simulink model "nlin_1DOF"  (R2025a)
settings: Solver=VariableStepAuto  StartTime=0.0  StopTime=50  RelTol=1e-3
settings Model: Creator=jidki  LastModifiedBy=jidki

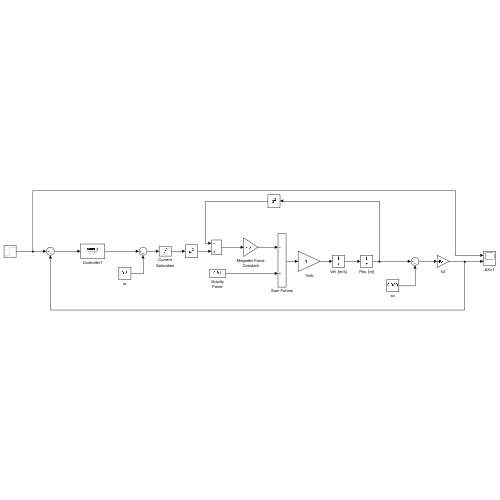
[thumbnail: Simulink's stored preview of the top-level diagram]
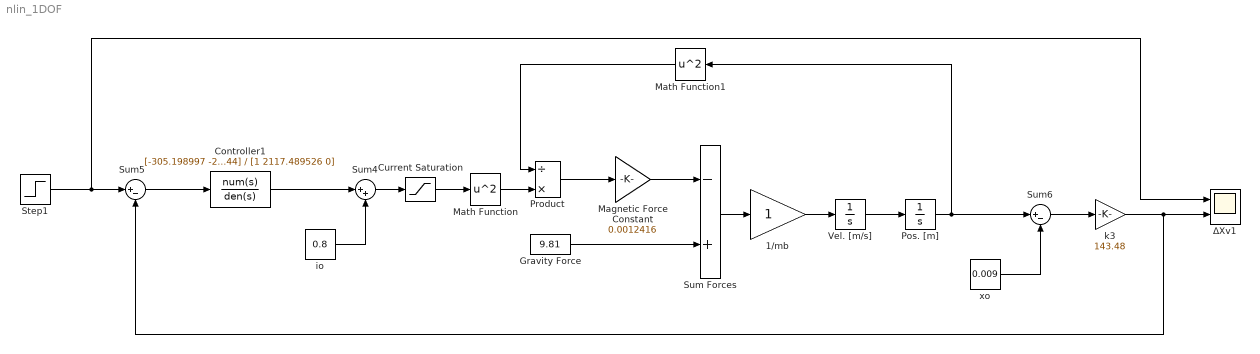
== system nlin_1DOF ==
  1/mb : Gain  SaturateOnIntegerOverflow=on  OutDataTypeStr=Inherit: Same as input  ParamDataTypeStr=Inherit: Same as input
  Controller1 : TransferFcn  Numerator=[-305.198997 -2531.996576 -2834.571544]  Denominator=[1 2117.489526 0]
  Current Saturation : Saturate  UpperLimit=1000  LowerLimit=-1000  ZeroCross=off
  Gravity Force : Constant  Value=9.81
  Magnetic Force Constant : Gain  Gain=0.0012416  SaturateOnIntegerOverflow=on  OutDataTypeStr=Inherit: Same as input  ParamDataTypeStr=Inherit: Same as input
  Math Function : Math  Operator=square  SignedPower=on
  Math Function1 : Math  Operator=square  SignedPower=on
  Pos. [m] : Integrator  InitialCondition=0.009  UpperSaturationLimit=0.005  LowerSaturationLimit=0  ZeroCross=off
  Product : Product  Inputs=/*  InputSameDT=on  SaturateOnIntegerOverflow=on  OutDataTypeStr=Inherit: Same as first input
  Step1 : Step  Time=25  After=143.48*0.009  SampleTime=0
  Sum Forces : Sum  Inputs=-+  InputSameDT=on  SaturateOnIntegerOverflow=on  OutDataTypeStr=Inherit: Same as first input
  Sum4 : Sum  Inputs=|++
  Sum5 : Sum  Inputs=|+-
  Sum6 : Sum  Inputs=|+-
  Vel. [m/s] : Integrator  UpperSaturationLimit=Inf  LowerSaturationLimit=-Inf  ZeroCross=off
  io : Constant  Value=0.8
  k3 : Gain  Gain=143.48
  xo : Constant  Value=0.009
  ΔXv1 : Scope  NumInputPorts=2
      settings: ActiveDisplayYMinimum=-1.3232219093615868E+9  ActiveDisplayYMaximum=1.1908997171341122E+10
  wires:
  Math Function1/1 -> Product/1
  Product/1 -> Magnetic Force Constant/1
  Gravity Force/1 -> Sum Forces/2
  Vel. [m/s]/1 -> Pos. [m]/1
  Sum Forces/1 -> 1/mb/1
  1/mb/1 -> Vel. [m/s]/1
  Current Saturation/1 -> Math Function/1
  Magnetic Force Constant/1 -> Sum Forces/1
  Math Function/1 -> Product/2
  Pos. [m]/1 -> Sum6/1, Math Function1/1
  Sum4/1 -> Current Saturation/1
  io/1 -> Sum4/2
  Controller1/1 -> Sum4/1
  Sum5/1 -> Controller1/1
  Sum6/1 -> k3/1
  k3/1 -> Sum5/2, ΔXv1/2
  Step1/1 -> ΔXv1/1, Sum5/1
  xo/1 -> Sum6/2
